simulink model "SeyyedAliSadat_DSTATCOM_FACTS_COURSE"  (R2022b)
settings: Solver=FixedStepDiscrete  StartTime=0.0  StopTime=3  FixedStep=Ts  RelTol=1e-3
InitFcn:
  |  Ts=5e-6;
undefined symbols (not defined in the file): D11, Delta, DiscIntNeverNeededParam
libraries: spsSeriesRLCBranchLib x9, spsGroundLib x6, spsThreePhaseVIMeasurementLib x4, spsSecondOrderFilterLib x4, slpidlib x4, spsLinearTransformerLib x3, spsVoltageMeasurementLib x3, spsThreePhaseParallelRLCLoadLib x2, spsUniversalBridgeLib x2, spsabctodq0Lib x2, spsPLL3phLib x2, spsPWMGenerator2LevelLib x2
(part 2 of 2)

== system SeyyedAliSadat_DSTATCOM_FACTS_COURSE/DStatcom/D_statcom Controller/Controller (sample time=Ts*32)/DC Voltage Regulator ==
  Vdc : Inport
  Vdc_Ref : Inport  Port=2
  -1<Id<+1 : Saturate  UpperLimit=1  LowerLimit=-1
  2250<Vdc<3750 : Saturate  UpperLimit=3750  LowerLimit=2250
  Discrete PI Controller : slpidlib/PID Controller  Controller=PI  Form=Parallel  TimeDomain=Discrete-time  UseExternalTs=off  SampleTime=Ts  IntegratorMethod=Forward Euler  FilterMethod=Forward Euler  ControllerParametersSource=internal  P=Kp  I=Ki  UseKiTs=off  D=0  N=100  UseFilter=on  TunerSelectOption=Transfer Function Based (PID Tuner App)  InitialConditionSource=internal  InitialConditionForIntegrator=0  InitialConditionForFilter=0  DifferentiatorICPrevScaledInput=0  ExternalReset=none  TrackingMode=off  Kt=1  LimitOutput=on  SatLimitsSource=internal  UpperSaturationLimit=1  LowerSaturationLimit=-1  LinearizeAsGain=off  AntiWindupMode=clamping  Kb=1  LimitIntegrator=off  UpperIntegratorSaturationLimit=inf  LowerIntegratorSaturationLimit=-inf  POutMin=[]  POutMax=[]  IOutMin=[]  IOutMax=[]  DOutMin=[]  DOutMax=[]  NOutMin=[]  NOutMax=[]  SumOutMin=[]  SumOutMax=[]  SaturationOutMin=[]  SaturationOutMax=[]  PParamMin=[]  PParamMax=[]  IParamMin=[]  IParamMax=[]  DParamMin=[]  DParamMax=[]  NParamMin=[]  NParamMax=[]  KbParamMin=[]  KbParamMax=[]  KtParamMin=[]  KtParamMax=[]  KbOutMin=[]  KbOutMax=[]  KtOutMin=[]  KtOutMax=[]  IntegratorOutMin=[]  IntegratorOutMax=[]  FilterOutMin=[]  FilterOutMax=[]  SumI1OutMin=[]  SumI1OutMax=[]  SumI2OutMin=[]  SumI2OutMax=[]  SumI3OutMin=[]  SumI3OutMax=[]  SumI4OutMin=[]  SumI4OutMax=[]  SumDOutMin=[]  SumDOutMax=[]  DifferentiatorOutMin=[]  DifferentiatorOutMax=[]  FilterDiffOutCoefMin=[]  FilterDiffOutCoefMax=[]  ReciprocalOutMin=[]  ReciprocalOutMax=[]  SumDenOutMin=[]  SumDenOutMax=[]  SumNumOutMin=[]  SumNumOutMax=[]  DivideOutMin=[]  DivideOutMax=[]  UdiffTsProdOutMin=[]  UdiffTsProdOutMax=[]  NTsProdOutMin=[]  NTsProdOutMax=[]  UintegralTsProdOutMin=[]  UintegralTsProdOutMax=[]  UngainTsProdOutMin=[]  UngainTsProdOutMax=[]  ClampingZeroOutDataTypeStr=Inherit: Inherit via back propagation  ClampingZeroOutMin=[]  ClampingZeroOutMax=[]  FilterDenConstantOutDataTypeStr=Inherit: Inherit via back propagation  FilterDenConstantOutMin=[]  FilterDenConstantOutMax=[]  PCopyOutDataTypeStr=Inherit: Inherit via back propagation  PCopyOutMin=[]  PCopyOutMax=[]  NCopyOutDataTypeStr=Inherit: Inherit via back propagation  NCopyOutMin=[]  NCopyOutMax=[]  IntegratorContinuousStateAttributes=''  IntegratorStateMustResolveToSignalObject=off  IntegratorRTWStateStorageClass=Auto  FilterContinuousStateAttributes=''  FilterStateMustResolveToSignalObject=off  FilterRTWStateStorageClass=Auto  ParallelPVariant=InternalParameters  IdealPVariant=Disabled  IVariant=InternalParameters  DVariant=Disabled  IntegratorVariant=Discrete  SatVariant=Enabled  AWVariant=DiscClampingParallel  PCopyVariant=Disabled  TRVariant=Disabled  FdbkBlocksVariant=Forward  IdealPFdbkVariant=Disabled  SatFdbkVariant=Disabled  DerivativeFilterVariant=Disabled  NVariant=Disabled  NCopyVariant=Disabled_SignalSpec  FilterICVariant=Disabled  IntegratorICVariant=InternalICs  ExternalResetVariant=Disabled  TRSumVariant=Passthrough  SumFdbkVariant=Disabled  SumVariant=Sum_PI  TsampFilterVariant=InternalTs  TsampNgainVariant=Passthrough  TsampIntegralVariant=Passthrough  ExternalSaturationOutDataTypeStr=Inherit: Same as second input
      settings: AttributesFormatString=P = %<P>\nI = %<I>
  Rate Limiter : RateLimiter  RisingSlewLimit=10000  FallingSlewLimit=-10000  SampleTimeMode=inherited  InitialCondition=3000
      settings: AttributesFormatString=Up = %<RisingSlewLimit>\nDown = %<FallingSlewLimit>\nIC = %<InitialCondition>
  Sum : Sum  Inputs=|+-  InputSameDT=on  SaturateOnIntegerOverflow=on  OutDataTypeStr=Inherit: Same as first input
  Id_Ref : Outport  InitialOutput=0
  wires:
  Discrete PI Controller/1 -> -1<Id<+1/1
  Sum/1 -> Discrete PI Controller/1
  -1<Id<+1/1 -> Id_Ref/1
  Rate Limiter/1 -> Sum/1
  Vdc/1 -> Sum/2
  2250<Vdc<3750/1 -> Rate Limiter/1
  Vdc_Ref/1 -> 2250<Vdc<3750/1

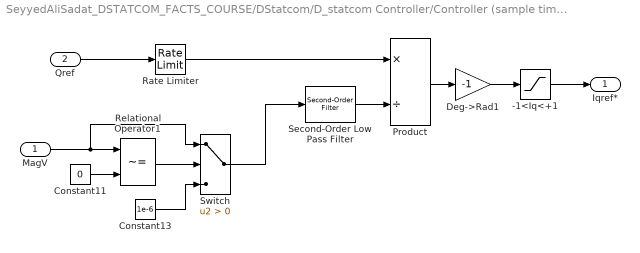
== system SeyyedAliSadat_DSTATCOM_FACTS_COURSE/DStatcom/D_statcom Controller/Controller (sample time=Ts*32)/Iq_ref (Manual) ==
  MagV : Inport  PortDimensions=1
  Qref : Inport  Port=2  PortDimensions=1
  -1<Iq<+1 : Saturate  UpperLimit=1  LowerLimit=-1
  Constant11 : Constant  Value=0
  Constant13 : Constant  Value=1e-6
  Deg->Rad1 : Gain  Gain=-1  SaturateOnIntegerOverflow=on  OutDataTypeStr=Inherit: Same as input  ParamDataTypeStr=Inherit: Same as input
  Product : Product  Inputs=*/  InputSameDT=on  SaturateOnIntegerOverflow=on  OutDataTypeStr=Inherit: Same as first input
  Rate Limiter : RateLimiter  RisingSlewLimit=60*2  FallingSlewLimit=-60*2  SampleTimeMode=inherited
      settings: AttributesFormatString=Up = %<RisingSlewLimit>\nDown = %<FallingSlewLimit>
  Relational Operator1 : RelationalOperator  Operator=~=
  Second-Order Low Pass Filter : spsSecondOrderFilterLib/Second-Order Filter  FilterType=Lowpass  Fo=20  Zeta=0.707  Ts=32*Ts  Initialize=off  Vac_Init="[0,  0,  60]"  Vdc_Init=0  PlotResponse=off  FreqRange=[0, 500, 1]
      settings: AttributesFormatString=f0: %<Fo>
      settings: LibrarySourceBlock=|
      | sps_lib/Control/Filters/Second-Order
      | Filter
  Switch : Switch  Criteria=u2 > Threshold
  Iqref* : Outport
  wires:
  Switch/1 -> Second-Order Low Pass Filter/1
  Second-Order Low Pass Filter/1 -> Product/2
  Constant11/1 -> Relational Operator1/2
  Relational Operator1/1 -> Switch/2
  MagV/1 -> Relational Operator1/1, Switch/1
  Constant13/1 -> Switch/3
  Product/1 -> Deg->Rad1/1
  Deg->Rad1/1 -> -1<Iq<+1/1
  -1<Iq<+1/1 -> Iqref*/1
  Qref/1 -> Rate Limiter/1
  Rate Limiter/1 -> Product/1

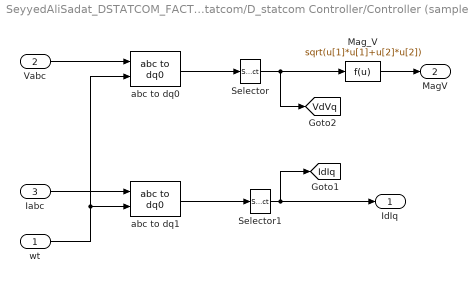
== system SeyyedAliSadat_DSTATCOM_FACTS_COURSE/DStatcom/D_statcom Controller/Controller (sample time=Ts*32)/Measuremnt Unit ==
  wt : Inport
  Vabc : Inport  Port=2
  Iabc : Inport  Port=3
  "Mag_V " : Fcn  Expr=sqrt(u[1]*u[1]+u[2]*u[2])
  Selector : Selector  InputPortWidth=3  IndexOptions=Index vector (dialog)  Indices=[1 2]  OutputSizes=1
  Selector1 : Selector  InputPortWidth=3  IndexOptions=Index vector (dialog)  Indices=[1 2]  OutputSizes=1
  abc to dq0 : spsabctodq0Lib/abc to dq0  Alignment=90 degrees behind phase A axis
  abc to dq1 : spsabctodq0Lib/abc to dq0  Alignment=90 degrees behind phase A axis
  IdIq : Outport
  MagV : Outport  Port=2
  tag scope: IdIq=global, VdVq=global
  wires:
  wt/1 -> abc to dq0/2, abc to dq1/2
  Vabc/1 -> abc to dq0/1
  abc to dq0/1 -> Selector/1
  Iabc/1 -> abc to dq1/1
  abc to dq1/1 -> Selector1/1
  Selector/1 -> [VdVq], "Mag_V "/1
  Selector1/1 -> IdIq/1, [IdIq]
  "Mag_V "/1 -> MagV/1

== system SeyyedAliSadat_DSTATCOM_FACTS_COURSE/DStatcom/D_statcom Controller/Controller (sample time=Ts*32)/Vd_Vq--> m,Phi ==
  VdVq : Inport
  Fcn3 : Fcn  Expr=sqrt(u[1]*u[1]+u[2]*u[2])
  Fcn4 : Fcn  Expr=atan2(u[2]+1e-6,u[1])*180/pi
  Mux2 : Mux  Inputs=2
  m_Phi : Outport
  wires:
  VdVq/1 -> Fcn3/1, Fcn4/1
  Fcn3/1 -> Mux2/1
  Mux2/1 -> m_Phi/1
  Fcn4/1 -> Mux2/2
